simulink model "blockdemo"  (Simulink 6.3)
settings: Solver=VariableStepDiscrete  StartTime=0.0  StopTime=1000  MaxStep=1  RelTol=1e-3
InitFcn:
  | %% DSPBuilder Start
  | alt_dspbuilder_update_model(bdroot)
  | %% DSPBuilder End
libraries: allblocks_alteradspbuilder2 x8
settings Model: Creator=mjervis  LastModifiedBy=delphick
settings OptimizationCC: BlockReduction=off  BooleanDataType=off  InlineInvariantSignals=on
settings DebuggingCC: SolverPrmCheckMsg=none
settings HardwareCC: TargetUnknown=on

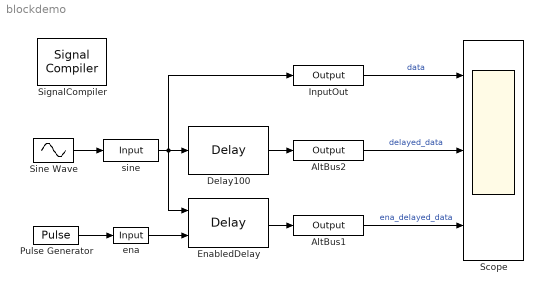
== system blockdemo ==
  AltBus1 : allblocks_alteradspbuilder2/Output  iofile=C:\workspace_clean\Documentation\DesignExamples\Tutorials\UnitBlocks\Storage\Delay\tb_blockdemo\blockdemo_AltBus1.capture  BusType=Signed Fractional  bwl=16  bwr=16  PORTTYPE=Output
  AltBus2 : allblocks_alteradspbuilder2/Output  iofile=C:\workspace_clean\Documentation\DesignExamples\Tutorials\UnitBlocks\Storage\Delay\tb_blockdemo\blockdemo_AltBus2.capture  BusType=Signed Fractional  bwl=16  bwr=16  PORTTYPE=Output
  Delay100 : allblocks_alteradspbuilder2/Delay  pipeline=100  ClockPhase=1  use_ena=off  use_sclr=off
  EnabledDelay : allblocks_alteradspbuilder2/Delay  pipeline=100  ClockPhase=1  use_ena=on  use_sclr=off
  InputOut : allblocks_alteradspbuilder2/Output  iofile=C:\workspace_clean\Documentation\DesignExamples\Tutorials\UnitBlocks\Storage\Delay\tb_blockdemo\blockdemo_InputOut.capture  BusType=Signed Fractional  bwl=16  bwr=16  PORTTYPE=Output
  Pulse Generator : DiscretePulseGenerator  Period=400  PulseWidth=200
      settings: AttributesFormatString=Period = %<Period>\nWidth = %<PulseWidth>
  Scope : Scope  NumInputPorts=3
      settings: TimeRange=1000  YMin=-50000~-50000~0  YMax=50000~50000~40000
  SignalCompiler : allblocks_alteradspbuilder2/Signal Compiler  DeviceFamily=Stratix III  DeviceName=AUTO  EnableSignalTap=off  SignalTapDepth=128  UseBoardBlock=off  StpUseDefaultClock=on  StpClock=clock
  Sine Wave : Sin  SineType=Sample based  Amplitude=(2^15)-1  Frequency=0.2  Samples=400  SampleTime=1
      settings: AttributesFormatString=Samples = %<Samples>\nAmplitude = %<Amplitude>
  ena : allblocks_alteradspbuilder2/Input  iofile=C:\workspace_clean\Documentation\DesignExamples\Tutorials\UnitBlocks\Storage\Delay\tb_blockdemo\blockdemo_ena.salt  BusType=Single Bit  bwl=16  bwr=16  SpecifyClock=off  PORTTYPE=Input
  sine : allblocks_alteradspbuilder2/Input  iofile=C:\workspace_clean\Documentation\DesignExamples\Tutorials\UnitBlocks\Storage\Delay\tb_blockdemo\blockdemo_sine.salt  BusType=Signed Fractional  bwl=16  bwr=16  SpecifyClock=off  PORTTYPE=Input
  wires:
  AltBus1/1 -> Scope/3  "ena_delayed_data"
  EnabledDelay/1 -> AltBus1/1
  Sine Wave/1 -> sine/1
  sine/1 -> EnabledDelay/1, InputOut/1, Delay100/1
  InputOut/1 -> Scope/1  "data"
  ena/1 -> EnabledDelay/2
  Pulse Generator/1 -> ena/1
  Delay100/1 -> AltBus2/1
  AltBus2/1 -> Scope/2  "delayed_data"
